simulink model "test_sim_2"  (R2022b)
settings: Solver=VariableStepAuto  StartTime=0.0  StopTime=10.0  RelTol=1e-3
undefined symbols (not defined in the file): tau1, tau2
settings Model: Creator=user  LastModifiedBy=user

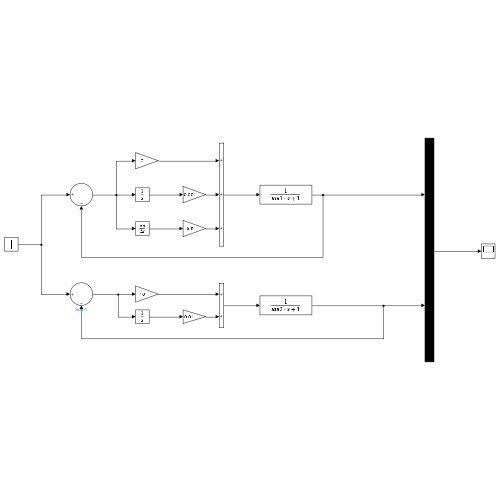
[thumbnail: Simulink's stored preview of the top-level diagram]
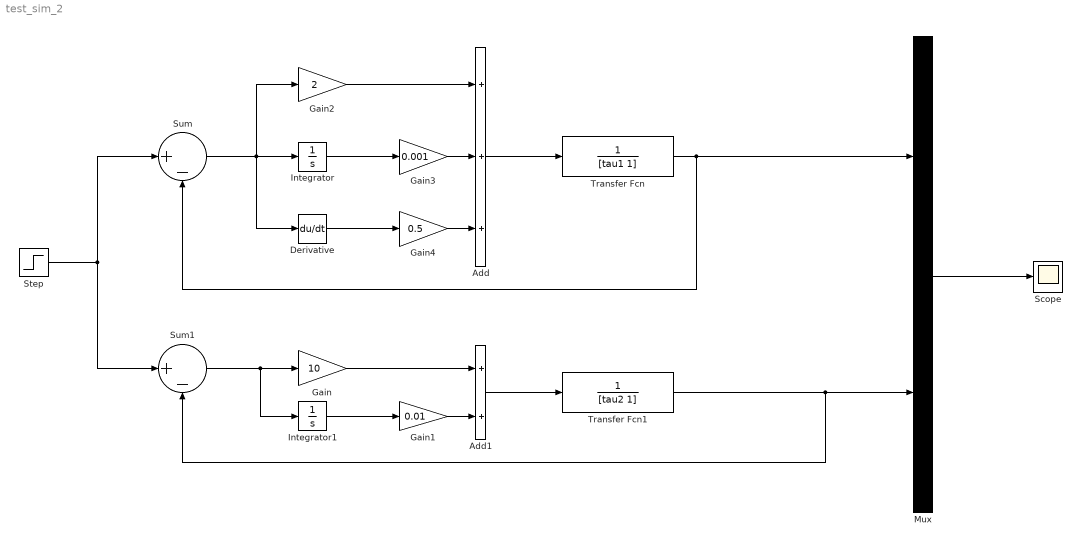
== system test_sim_2 ==
  Add : Sum  Inputs=+++
  Add1 : Sum
  Derivative : Derivative
  Gain : Gain  Gain=10
  Gain1 : Gain  Gain=0.01
  Gain2 : Gain  Gain=2
  Gain3 : Gain  Gain=0.001
  Gain4 : Gain  Gain=0.5
  Integrator : Integrator
  Integrator1 : Integrator
  Mux : Mux  Inputs=2
  Scope : Scope
  Step : Step  Before=60  After=100  SampleTime=0
  Sum : Sum  Inputs=|+-
  Sum1 : Sum  Inputs=|+-
  Transfer Fcn : TransferFcn  Denominator=[tau1 1]
  Transfer Fcn1 : TransferFcn  Denominator=[tau2 1]
  wires:
  Step/1 -> Sum/1, Sum1/1
  Sum/1 -> Gain2/1, Derivative/1, Integrator/1
  Sum1/1 -> Integrator1/1, Gain/1
  Integrator/1 -> Gain3/1
  Gain3/1 -> Add/2
  Gain2/1 -> Add/1
  Add/1 -> Transfer Fcn/1
  Integrator1/1 -> Gain1/1
  Gain1/1 -> Add1/2
  Gain/1 -> Add1/1
  Add1/1 -> Transfer Fcn1/1
  Transfer Fcn/1 -> Sum/2, Mux/1
  Transfer Fcn1/1 -> Sum1/2, Mux/2
  Mux/1 -> Scope/1
  Derivative/1 -> Gain4/1
  Gain4/1 -> Add/3
